simulink model "sm_test_wout_simmech"  (R2020a)
settings: Solver=ode45  StartTime=0.0  StopTime=100  RelTol=1e-20  EnableMultiTasking=on
values from neighbouring files (symbols this model uses):
  g = 9.81    [run_wout_simmech.m]
  k = 0    [run_wout_simmech.m]
  l1 = 1    [run_wout_simmech.m]
  m = 15    [run_wout_simmech.m]
  M = 5    [run_wout_simmech.m]
  r0 = 0    [run_wout_simmech.m]
  theta0 = deg2rad(5)    [run_wout_simmech.m]
settings Model: Creator=Zdenek Boucek  LastModifiedBy=Jiří
settings DataIOCC: LimitDataPoints=on  SaveFormat=Array  SignalLoggingSaveFormat=ModelDataLogs  ReturnWorkspaceOutputs=off
settings OptimizationCC: ExpressionDepthLimit=2147483647  LifeSpan=inf
settings DebuggingCC: UnderspecifiedInitializationDetection=Classic  MergeDetectMultiDrivingBlocksExec=none  SolverPrmCheckMsg=warning  FcnCallInpInsideContextMsg=warning  StateNameClashWarn=warning  SFUnexpectedBacktrackingDiag=warning  SFNoUnconditionalDefaultTransitionDiag=warning  SFExecutionAtInitializationDiag=none  ArithmeticOperatorsInVariantConditions=warning
settings HardwareCC: ProdBitPerPointer=32  ProdBitPerSizeT=32  ProdBitPerPtrDiffT=32  ProdLargestAtomicFloat=None  ProdIntDivRoundTo=Undefined  ProdEndianess=Unspecified  ProdWordSize=32  ProdHWDeviceType=32-bit Generic
settings ModelReferenceCC: PropagateSignalLabelsOutOfModel=off
settings SFSimCC: SimUseLocalCustomCode=off  CustomCodeUndefinedFunction=UseInterfaceOnly
settings RTWCC: RTWUseLocalCustomCode=off
settings CodeAppCC: StateflowObjectComments=on
settings GRTTargetCC: TargetLangStandard=C89/C90 (ANSI)  CombineOutputUpdateFcns=off  GRTInterface=on
settings ConfigComp: CovMetricSettings=dw  CovHtmlReporting=on  CovSaveCumulativeToWorkspaceVar=on  CovSaveSingleToWorkspaceVar=on  CovExternalEMLEnable=off
settings SimscapeCC: SimscapeNormalizeSystem=off
settings ConfigurationSet: Description=SimMechanics 2G

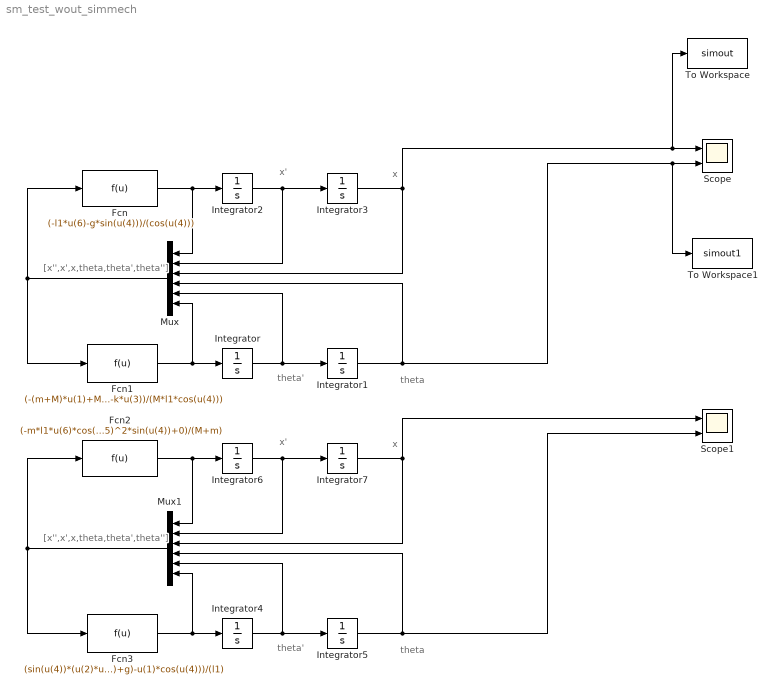
== system sm_test_wout_simmech ==
  note: x'
  note: x
  note: theta'
  note: theta
  note: [x'',x',x,theta,theta',theta'']
  note: x'
  note: x
  note: theta'
  note: theta
  note: [x'',x',x,theta,theta',theta'']
  Fcn : Fcn  Expr=(-l1*u(6)-g*sin(u(4)))/(cos(u(4)))
  Fcn1 : Fcn  Expr=(-(m+M)*u(1)+M*l1*u(5)*u(5)*sin(u(4))-k*u(3))/(M*l1*cos(u(4)))
  Fcn2 : Fcn  Expr=(-m*l1*u(6)*cos(u(4))+m*l1*u(5)^2*sin(u(4))+0)/(M+m)
  Fcn3 : Fcn  Expr=(sin(u(4))*(u(2)*u(5)-u(2)+g)-u(1)*cos(u(4)))/(l1)
  Integrator{,2,4,6} (4 alike) : Integrator
  Integrator1 : Integrator  InitialCondition=theta0
  Integrator3 : Integrator  InitialCondition=r0
  Integrator5 : Integrator  InitialCondition=theta0
  Integrator7 : Integrator  InitialCondition=r0
  Mux : Mux  Inputs=6
  Mux1 : Mux  Inputs=6
  Scope : Scope  NumInputPorts=2
  Scope1 : Scope  NumInputPorts=2
  To Workspace : ToWorkspace  VariableName=simout  SaveFormat=Structure With Time  SampleTime=-1
  To Workspace1 : ToWorkspace  VariableName=simout1  SaveFormat=Structure With Time  SampleTime=-1
  wires:
  Fcn/1 -> Integrator2/1, Mux/1
  Integrator2/1 -> Integrator3/1, Mux/2
  Fcn1/1 -> Integrator/1, Mux/6
  Integrator/1 -> Integrator1/1, Mux/5
  Mux/1 -> Fcn1/1, Fcn/1
  Integrator1/1 -> Scope/2, To Workspace1/1, Mux/4
  Integrator3/1 -> Scope/1, To Workspace/1, Mux/3
  Integrator7/1 -> Scope1/1, Mux1/3
  Integrator5/1 -> Mux1/4, Scope1/2
  Mux1/1 -> Fcn2/1, Fcn3/1
  Integrator4/1 -> Mux1/5, Integrator5/1
  Fcn3/1 -> Mux1/6, Integrator4/1
  Integrator6/1 -> Mux1/2, Integrator7/1
  Fcn2/1 -> Mux1/1, Integrator6/1
